simulink model "CMOS_Kernel_Memory_Sync"  (R2023b)
settings: Solver=VariableStepAuto  StartTime=0.0  StopTime=30000000  RelTol=1e-3
values from neighbouring files (symbols this model uses):
  AmountOfPixelsPerScanline = 400    [Kernel_Setup_Script.m]
  AmountOfRamBlocksScanlines = 5    [Kernel_Setup_Script.m]
  AmountOfRamBlocksScanlinesOffset = AmountOfRamBlocksScanlines - 1    (= 4)    [Kernel_Setup_Script.m]
  AmountOfScanlinePixels = 73700    [Kernel_Setup_Script.m]
  AmountOfScanlinePixelsOffset = AmountOfScanlinePixels - 1    (= 73699)    [Kernel_Setup_Script.m]
  AmountOfScanlines = 1100    [Kernel_Setup_Script.m]
  AmountOfScanlinesOffset = AmountOfScanlines - 1    (= 1099)    [Kernel_Setup_Script.m]
  AOPPK_Off = AmountOfPixelsPerScanline - 1    (= 399)    [Kernel_Setup_Script.m]
  AOPPS_Off = AmountOfPixelsPerScanline - 1    (= 399)    [Kernel_Setup_Script.m]
  FramePackOff_0 = FramePackOff_0 - ScanlineFifoCheck    [Kernel_Setup_Script.m]
  FramePackOff_1 = FramePackOff_1 - ScanlineFifoCheck    [Kernel_Setup_Script.m]
  FramePackOff_2 = FramePackOff_2 - ScanlineFifoCheck    [Kernel_Setup_Script.m]
  FramePackOff_3 = FramePackOff_3 - ScanlineFifoCheck    [Kernel_Setup_Script.m]
  FramePackOff_4 = FramePackOff_4 - ScanlineFifoCheck    [Kernel_Setup_Script.m]
  FramePackOff_5 = FramePackOff_5 - ScanlineFifoCheck    [Kernel_Setup_Script.m]
  KernelPackOff_0 = KernelPackOff_0 - KernelBitsPerRow    [Kernel_Setup_Script.m]
  KernelPackOff_1 = KernelPackOff_1 - KernelBitsPerRow    [Kernel_Setup_Script.m]
  KernelPackOff_2 = KernelPackOff_2 - KernelBitsPerRow    [Kernel_Setup_Script.m]
  KernelPackOff_3 = KernelPackOff_3 - KernelBitsPerRow    [Kernel_Setup_Script.m]
  Slice59DownTo48Top = (MsbOffset - (ScanlinePixelBitSizeController*1))    (= 59)    [Kernel_Setup_Script.m]
  Slice71DownTo60Top = (MsbOffset - (ScanlinePixelBitSizeController*0))    (= 71)    [Kernel_Setup_Script.m]
  TotalSectionsForFrames = AmountOfScanlines/AmountOfRamBlocksScanlines    (= 220)    [Kernel_Setup_Script.m]
  UltraRamRows = AmountOfPixelsPerScanline/ScanlineFifoCheck    [Kernel_Setup_Script.m]
  UltraRamRowsCeil = ceil(AmountOfPixelsPerScanline/ScanlineFifoCheck)    [Kernel_Setup_Script.m]
  UltraRamRowsKernel = AmountOfPixelsPerScanline/KernelBitsPerRow    (= 100)    [Kernel_Setup_Script.m]
  UltraRamRowsKernelCeil = ceil(AmountOfPixelsPerScanline/KernelBitsPerRow)    [Kernel_Setup_Script.m]
  UltraRamRowsMemorySectionOffset = UltraRamRowsCeil*AmountOfRamBlocksScanlines    [Kernel_Setup_Script.m]
  UltraRamRowsOffset = UltraRamRowsCeil - 1    [Kernel_Setup_Script.m]
undefined symbols (not defined in the file or in its folder): c, Down, sfvc784, Up, xck26
libraries: hdlBasic x4512, vmcUtilities x1
(part 3 of 39)

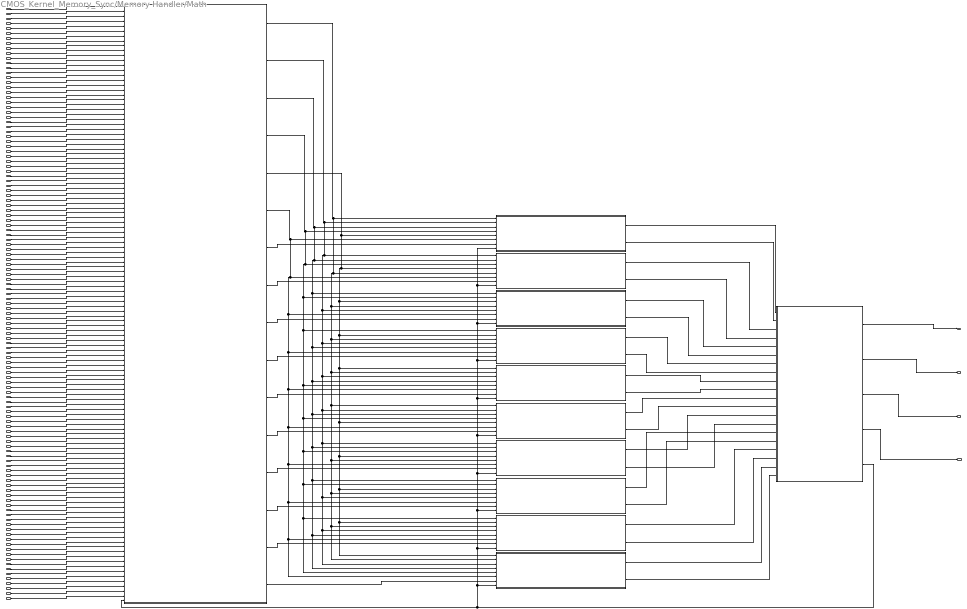
== system CMOS_Kernel_Memory_Sync/Memory Handler/Math ==
  In Pixel 0 at Offset 0 : Inport
  In Pixel 1 at Offset 0 : Inport  Port=2
  In Pixel 2 at Offset 0 : Inport  Port=3
  In Pixel 3 at Offset 0 : Inport  Port=4
  In Pixel 4 at Offset 0 : Inport  Port=5
  In Pixel 5 at Offset 0 : Inport  Port=6
  In Pixel 6 at Offset 0 : Inport  Port=7
  In Pixel 7 at Offset 0 : Inport  Port=8
  In Pixel 8 at Offset 0 : Inport  Port=9
  In Pixel 9 at Offset 0 : Inport  Port=10
  In Pixel 10 at Offset 0 : Inport  Port=11
  In Pixel 11 at Offset 0 : Inport  Port=12
  In Pixel 0 at Offset 1 : Inport  Port=13
  In Pixel 1 at Offset 1 : Inport  Port=14
  In Pixel 2 at Offset 1 : Inport  Port=15
  In Pixel 3 at Offset 1 : Inport  Port=16
  In Pixel 4 at Offset 1 : Inport  Port=17
  In Pixel 5 at Offset 1 : Inport  Port=18
  In Pixel 6 at Offset 1 : Inport  Port=19
  In Pixel 7 at Offset 1 : Inport  Port=20
  In Pixel 8 at Offset 1 : Inport  Port=21
  In Pixel 9 at Offset 1 : Inport  Port=22
  In Pixel 10 at Offset 1 : Inport  Port=23
  In Pixel 11 at Offset 1 : Inport  Port=24
  In Pixel 0 at Offset 2 : Inport  Port=25
  In Pixel 1 at Offset 2 : Inport  Port=26
  In Pixel 2 at Offset 2 : Inport  Port=27
  In Pixel 3 at Offset 2 : Inport  Port=28
  In Pixel 4 at Offset 2 : Inport  Port=29
  In Pixel 5 at Offset 2 : Inport  Port=30
  In Pixel 6 at Offset 2 : Inport  Port=31
  In Pixel 7 at Offset 2 : Inport  Port=32
  In Pixel 8 at Offset 2 : Inport  Port=33
  In Pixel 9 at Offset 2 : Inport  Port=34
  In Pixel 10 at Offset 2 : Inport  Port=35
  In Pixel 11 at Offset 2 : Inport  Port=36
  In Pixel 0 at Offset 3 : Inport  Port=37
  In Pixel 1 at Offset 3 : Inport  Port=38
  In Pixel 2 at Offset 3 : Inport  Port=39
  In Pixel 3 at Offset 3 : Inport  Port=40
  In Pixel 4 at Offset 3 : Inport  Port=41
  In Pixel 5 at Offset 3 : Inport  Port=42
  In Pixel 6 at Offset 3 : Inport  Port=43
  In Pixel 7 at Offset 3 : Inport  Port=44
  In Pixel 8 at Offset 3 : Inport  Port=45
  In Pixel 9 at Offset 3 : Inport  Port=46
  In Pixel 10 at Offset 3 : Inport  Port=47
  In Pixel 11 at Offset 3 : Inport  Port=48
  In Pixel 0 at Offset 4 : Inport  Port=49
  In Pixel 1 at Offset 4 : Inport  Port=50
  In Pixel 2 at Offset 4 : Inport  Port=51
  In Pixel 3 at Offset 4 : Inport  Port=52
  In Pixel 4 at Offset 4 : Inport  Port=53
  In Pixel 5 at Offset 4 : Inport  Port=54
  In Pixel 6 at Offset 4 : Inport  Port=55
  In Pixel 7 at Offset 4 : Inport  Port=56
  In Pixel 8 at Offset 4 : Inport  Port=57
  In Pixel 9 at Offset 4 : Inport  Port=58
  In Pixel 10 at Offset 4 : Inport  Port=59
  In Pixel 11 at Offset 4 : Inport  Port=60
  In Weight 0 at Offset 0 : Inport  Port=61
  In Weight 1 at Offset 0 : Inport  Port=62
  In Weight 2 at Offset 0 : Inport  Port=63
  In Weight 3 at Offset 0 : Inport  Port=64
  In Weight 4 at Offset 0 : Inport  Port=65
  In Weight 5 at Offset 0 : Inport  Port=66
  In Weight 6 at Offset 0 : Inport  Port=67
  In Weight 7 at Offset 0 : Inport  Port=68
  In Weight 8 at Offset 0 : Inport  Port=69
  In Weight 9 at Offset 0 : Inport  Port=70
  In Weight 10 at Offset 0 : Inport  Port=71
  In Weight 11 at Offset 0 : Inport  Port=72
  In Weight 0 at Offset 1 : Inport  Port=73
  In Weight 1 at Offset 1 : Inport  Port=74
  In Weight 2 at Offset 1 : Inport  Port=75
  In Weight 3 at Offset 1 : Inport  Port=76
  In Weight 4 at Offset 1 : Inport  Port=77
  In Weight 5 at Offset 1 : Inport  Port=78
  In Weight 6 at Offset 1 : Inport  Port=79
  In Weight 7 at Offset 1 : Inport  Port=80
  In Weight 8 at Offset 1 : Inport  Port=81
  In Weight 9 at Offset 1 : Inport  Port=82
  In Weight 10 at Offset 1 : Inport  Port=83
  In Weight 11 at Offset 1 : Inport  Port=84
  In Weight 0 at Offset 2 : Inport  Port=85
  In Weight 1 at Offset 2 : Inport  Port=86
  In Weight 2 at Offset 2 : Inport  Port=87
  In Weight 3 at Offset 2 : Inport  Port=88
  In Weight 4 at Offset 2 : Inport  Port=89
  In Weight 5 at Offset 2 : Inport  Port=90
  In Weight 6 at Offset 2 : Inport  Port=91
  In Weight 7 at Offset 2 : Inport  Port=92
  In Weight 8 at Offset 2 : Inport  Port=93
  In Weight 9 at Offset 2 : Inport  Port=94
  In Weight 10 at Offset 2 : Inport  Port=95
  In Weight 11 at Offset 2 : Inport  Port=96
  In Weight 0 at Offset 3 : Inport  Port=97
  In Weight 1 at Offset 3 : Inport  Port=98
  In Weight 2 at Offset 3 : Inport  Port=99
  In Weight 3 at Offset 3 : Inport  Port=100
  In Weight 4 at Offset 3 : Inport  Port=101
  In Weight 5 at Offset 3 : Inport  Port=102
  In Weight 6 at Offset 3 : Inport  Port=103
  In Weight 7 at Offset 3 : Inport  Port=104
  In Weight 8 at Offset 3 : Inport  Port=105
  In Weight 9 at Offset 3 : Inport  Port=106
  In Weight 10 at Offset 3 : Inport  Port=107
  In Weight 11 at Offset 3 : Inport  Port=108
  In Weight 0 at Offset 4 : Inport  Port=109
  In Weight 1 at Offset 4 : Inport  Port=110
  In Weight 2 at Offset 4 : Inport  Port=111
  In Weight 3 at Offset 4 : Inport  Port=112
  In Weight 4 at Offset 4 : Inport  Port=113
  In Weight 5 at Offset 4 : Inport  Port=114
  In Weight 6 at Offset 4 : Inport  Port=115
  In Weight 7 at Offset 4 : Inport  Port=116
  In Weight 8 at Offset 4 : Inport  Port=117
  In Weight 9 at Offset 4 : Inport  Port=118
  In Weight 10 at Offset 4 : Inport  Port=119
  In Weight 11 at Offset 4 : Inport  Port=120
  Valid Data In : Inport  Port=121
  Kernel Organizer : Subsystem
  Kernel Result 0 : Subsystem
  Kernel Result 1 : Subsystem
  Kernel Result 2 : Subsystem
  Kernel Result 3 : Subsystem
  Kernel Result 4 : Subsystem
  Kernel Result 5 : Subsystem
  Kernel Result 6 : Subsystem
  Kernel Result 7 : Subsystem
  Kernel Result 8 : Subsystem
  Kernel Result 9 : Subsystem
  Subsystem : Subsystem
  Kernel Output : Outport
  Valid Kernel Output : Outport  Port=2
  Kernel Result Array Position : Outport  Port=3
  Kernel Result Row Depth Position : Outport  Port=4
  wires:
  Kernel Organizer/1(Pixel Group Offset 0) -> Kernel Result 0/1(Pixel Bus Input Offset 0), Kernel Result 2/4(Pixel Bus Input Offset 3), Kernel Result 3/3(Pixel Bus Input Offset 2), Kernel Result 4/2(Pixel Bus Input Offset 1), Kernel Result 5/1(Pixel Bus Input Offset 0), Kernel Result 6/5(Pixel Bus Input Offset 4), Kernel Result 7/4(Pixel Bus Input Offset 3), Kernel Result 9/2(Pixel Bus Input Offset 1), Kernel Result 8/3(Pixel Bus Input Offset 2), Kernel Result 1/5(Pixel Bus Input Offset 4)
  Kernel Organizer/7(Kernel Result Valid Bus 0) -> Kernel Result 0/7(Valid Bus Input)
  Valid Data In/1 -> Kernel Organizer/121(Valid Data In)
  In Weight 11 at Offset 4/1 -> Kernel Organizer/120(In Weight 11 at Offset 4)
  In Weight 10 at Offset 4/1 -> Kernel Organizer/119(In Weight 10 at Offset 4)
  In Weight 9 at Offset 4/1 -> Kernel Organizer/118(In Weight 9 at Offset 4)
  In Weight 8 at Offset 4/1 -> Kernel Organizer/117(In Weight 8 at Offset 4)
  In Weight 7 at Offset 4/1 -> Kernel Organizer/116(In Weight 7 at Offset 4)
  In Weight 6 at Offset 4/1 -> Kernel Organizer/115(In Weight 6 at Offset 4)
  In Weight 5 at Offset 4/1 -> Kernel Organizer/114(In Weight 5 at Offset 4)
  In Weight 4 at Offset 4/1 -> Kernel Organizer/113(In Weight 4 at Offset 4)
  In Weight 3 at Offset 4/1 -> Kernel Organizer/112(In Weight 3 at Offset 4)
  In Weight 2 at Offset 4/1 -> Kernel Organizer/111(In Weight 2 at Offset 4)
  In Weight 1 at Offset 4/1 -> Kernel Organizer/110(In Weight 1 at Offset 4)
  In Weight 0 at Offset 4/1 -> Kernel Organizer/109(In Weight 0 at Offset 4)
  In Weight 11 at Offset 3/1 -> Kernel Organizer/108(In Weight 11 at Offset 3)
  In Weight 10 at Offset 3/1 -> Kernel Organizer/107(In Weight 10 at Offset 3)
  In Weight 9 at Offset 3/1 -> Kernel Organizer/106(In Weight 9 at Offset 3)
  In Weight 8 at Offset 3/1 -> Kernel Organizer/105(In Weight 8 at Offset 3)
  In Weight 7 at Offset 3/1 -> Kernel Organizer/104(In Weight 7 at Offset 3)
  In Weight 6 at Offset 3/1 -> Kernel Organizer/103(In Weight 6 at Offset 3)
  In Weight 5 at Offset 3/1 -> Kernel Organizer/102(In Weight 5 at Offset 3)
  In Weight 4 at Offset 3/1 -> Kernel Organizer/101(In Weight 4 at Offset 3)
  In Weight 3 at Offset 3/1 -> Kernel Organizer/100(In Weight 3 at Offset 3)
  In Weight 2 at Offset 3/1 -> Kernel Organizer/99(In Weight 2 at Offset 3)
  In Weight 1 at Offset 3/1 -> Kernel Organizer/98(In Weight 1 at Offset 3)
  In Weight 0 at Offset 3/1 -> Kernel Organizer/97(In Weight 0 at Offset 3)
  In Weight 6 at Offset 2/1 -> Kernel Organizer/91(In Weight 6 at Offset 2)
  In Weight 5 at Offset 1/1 -> Kernel Organizer/78(In Weight 5 at Offset 1)
  In Weight 6 at Offset 1/1 -> Kernel Organizer/79(In Weight 6 at Offset 1)
  In Weight 5 at Offset 2/1 -> Kernel Organizer/90(In Weight 5 at Offset 2)
  In Weight 7 at Offset 1/1 -> Kernel Organizer/80(In Weight 7 at Offset 1)
  In Weight 8 at Offset 2/1 -> Kernel Organizer/93(In Weight 8 at Offset 2)
  In Weight 1 at Offset 2/1 -> Kernel Organizer/86(In Weight 1 at Offset 2)
  In Weight 1 at Offset 1/1 -> Kernel Organizer/74(In Weight 1 at Offset 1)
  In Weight 11 at Offset 2/1 -> Kernel Organizer/96(In Weight 11 at Offset 2)
  In Weight 10 at Offset 2/1 -> Kernel Organizer/95(In Weight 10 at Offset 2)
  In Weight 2 at Offset 1/1 -> Kernel Organizer/75(In Weight 2 at Offset 1)
  In Weight 9 at Offset 2/1 -> Kernel Organizer/94(In Weight 9 at Offset 2)
  In Weight 3 at Offset 2/1 -> Kernel Organizer/88(In Weight 3 at Offset 2)
  In Weight 8 at Offset 1/1 -> Kernel Organizer/81(In Weight 8 at Offset 1)
  In Weight 4 at Offset 1/1 -> Kernel Organizer/77(In Weight 4 at Offset 1)
  In Weight 0 at Offset 2/1 -> Kernel Organizer/85(In Weight 0 at Offset 2)
  In Weight 3 at Offset 1/1 -> Kernel Organizer/76(In Weight 3 at Offset 1)
  In Weight 10 at Offset 1/1 -> Kernel Organizer/83(In Weight 10 at Offset 1)
  In Weight 4 at Offset 2/1 -> Kernel Organizer/89(In Weight 4 at Offset 2)
  In Weight 9 at Offset 1/1 -> Kernel Organizer/82(In Weight 9 at Offset 1)
  In Weight 7 at Offset 2/1 -> Kernel Organizer/92(In Weight 7 at Offset 2)
  In Weight 11 at Offset 1/1 -> Kernel Organizer/84(In Weight 11 at Offset 1)
  In Weight 2 at Offset 2/1 -> Kernel Organizer/87(In Weight 2 at Offset 2)
  In Weight 6 at Offset 0/1 -> Kernel Organizer/67(In Weight 6 at Offset 0)
  In Pixel 5 at Offset 4/1 -> Kernel Organizer/54(In Pixel 5 at Offset 4)
  In Pixel 6 at Offset 4/1 -> Kernel Organizer/55(In Pixel 6 at Offset 4)
  In Weight 5 at Offset 0/1 -> Kernel Organizer/66(In Weight 5 at Offset 0)
  In Pixel 7 at Offset 4/1 -> Kernel Organizer/56(In Pixel 7 at Offset 4)
  In Weight 8 at Offset 0/1 -> Kernel Organizer/69(In Weight 8 at Offset 0)
  In Weight 1 at Offset 0/1 -> Kernel Organizer/62(In Weight 1 at Offset 0)
  In Pixel 1 at Offset 4/1 -> Kernel Organizer/50(In Pixel 1 at Offset 4)
  In Weight 11 at Offset 0/1 -> Kernel Organizer/72(In Weight 11 at Offset 0)
  In Weight 10 at Offset 0/1 -> Kernel Organizer/71(In Weight 10 at Offset 0)
  In Pixel 2 at Offset 4/1 -> Kernel Organizer/51(In Pixel 2 at Offset 4)
  In Weight 9 at Offset 0/1 -> Kernel Organizer/70(In Weight 9 at Offset 0)
  In Weight 3 at Offset 0/1 -> Kernel Organizer/64(In Weight 3 at Offset 0)
  In Pixel 8 at Offset 4/1 -> Kernel Organizer/57(In Pixel 8 at Offset 4)
  In Pixel 4 at Offset 4/1 -> Kernel Organizer/53(In Pixel 4 at Offset 4)
  In Weight 0 at Offset 0/1 -> Kernel Organizer/61(In Weight 0 at Offset 0)
  In Weight 0 at Offset 1/1 -> Kernel Organizer/73(In Weight 0 at Offset 1)
  In Pixel 3 at Offset 4/1 -> Kernel Organizer/52(In Pixel 3 at Offset 4)
  In Pixel 10 at Offset 4/1 -> Kernel Organizer/59(In Pixel 10 at Offset 4)
  In Weight 4 at Offset 0/1 -> Kernel Organizer/65(In Weight 4 at Offset 0)
  In Pixel 9 at Offset 4/1 -> Kernel Organizer/58(In Pixel 9 at Offset 4)
  In Weight 7 at Offset 0/1 -> Kernel Organizer/68(In Weight 7 at Offset 0)
  In Pixel 11 at Offset 4/1 -> Kernel Organizer/60(In Pixel 11 at Offset 4)
  In Weight 2 at Offset 0/1 -> Kernel Organizer/63(In Weight 2 at Offset 0)
  In Pixel 6 at Offset 3/1 -> Kernel Organizer/43(In Pixel 6 at Offset 3)
  In Pixel 5 at Offset 2/1 -> Kernel Organizer/30(In Pixel 5 at Offset 2)
  In Pixel 1 at Offset 0/1 -> Kernel Organizer/2(In Pixel 1 at Offset 0)
  In Pixel 5 at Offset 3/1 -> Kernel Organizer/42(In Pixel 5 at Offset 3)
  In Pixel 7 at Offset 2/1 -> Kernel Organizer/32(In Pixel 7 at Offset 2)
  In Pixel 1 at Offset 3/1 -> Kernel Organizer/38(In Pixel 1 at Offset 3)
  In Pixel 1 at Offset 2/1 -> Kernel Organizer/26(In Pixel 1 at Offset 2)
  In Pixel 11 at Offset 3/1 -> Kernel Organizer/48(In Pixel 11 at Offset 3)
  In Pixel 10 at Offset 3/1 -> Kernel Organizer/47(In Pixel 10 at Offset 3)
  In Pixel 9 at Offset 3/1 -> Kernel Organizer/46(In Pixel 9 at Offset 3)
  In Pixel 0 at Offset 0/1 -> Kernel Organizer/1(In Pixel 0 at Offset 0)
  In Pixel 1 at Offset 1/1 -> Kernel Organizer/14(In Pixel 1 at Offset 1)
  In Pixel 4 at Offset 1/1 -> Kernel Organizer/17(In Pixel 4 at Offset 1)
  In Pixel 8 at Offset 1/1 -> Kernel Organizer/21(In Pixel 8 at Offset 1)
  In Pixel 3 at Offset 1/1 -> Kernel Organizer/16(In Pixel 3 at Offset 1)
  In Pixel 2 at Offset 1/1 -> Kernel Organizer/15(In Pixel 2 at Offset 1)
  In Pixel 8 at Offset 3/1 -> Kernel Organizer/45(In Pixel 8 at Offset 3)
  In Pixel 10 at Offset 1/1 -> Kernel Organizer/23(In Pixel 10 at Offset 1)
  In Pixel 9 at Offset 1/1 -> Kernel Organizer/22(In Pixel 9 at Offset 1)
  In Pixel 10 at Offset 0/1 -> Kernel Organizer/11(In Pixel 10 at Offset 0)
  In Pixel 3 at Offset 3/1 -> Kernel Organizer/40(In Pixel 3 at Offset 3)
  In Pixel 4 at Offset 2/1 -> Kernel Organizer/29(In Pixel 4 at Offset 2)
  In Pixel 7 at Offset 1/1 -> Kernel Organizer/20(In Pixel 7 at Offset 1)
  In Pixel 2 at Offset 2/1 -> Kernel Organizer/27(In Pixel 2 at Offset 2)
  In Pixel 11 at Offset 0/1 -> Kernel Organizer/12(In Pixel 11 at Offset 0)
  In Pixel 11 at Offset 1/1 -> Kernel Organizer/24(In Pixel 11 at Offset 1)
  In Pixel 8 at Offset 0/1 -> Kernel Organizer/9(In Pixel 8 at Offset 0)
  In Pixel 0 at Offset 1/1 -> Kernel Organizer/13(In Pixel 0 at Offset 1)
  In Pixel 8 at Offset 2/1 -> Kernel Organizer/33(In Pixel 8 at Offset 2)
  In Pixel 4 at Offset 0/1 -> Kernel Organizer/5(In Pixel 4 at Offset 0)
  In Pixel 5 at Offset 1/1 -> Kernel Organizer/18(In Pixel 5 at Offset 1)
  In Pixel 6 at Offset 2/1 -> Kernel Organizer/31(In Pixel 6 at Offset 2)
  In Pixel 5 at Offset 0/1 -> Kernel Organizer/6(In Pixel 5 at Offset 0)
  In Pixel 6 at Offset 0/1 -> Kernel Organizer/7(In Pixel 6 at Offset 0)
  In Pixel 3 at Offset 0/1 -> Kernel Organizer/4(In Pixel 3 at Offset 0)
  In Pixel 9 at Offset 0/1 -> Kernel Organizer/10(In Pixel 9 at Offset 0)
  In Pixel 7 at Offset 0/1 -> Kernel Organizer/8(In Pixel 7 at Offset 0)
  In Pixel 0 at Offset 2/1 -> Kernel Organizer/25(In Pixel 0 at Offset 2)
  In Pixel 2 at Offset 0/1 -> Kernel Organizer/3(In Pixel 2 at Offset 0)
  In Pixel 0 at Offset 3/1 -> Kernel Organizer/37(In Pixel 0 at Offset 3)
  In Pixel 0 at Offset 4/1 -> Kernel Organizer/49(In Pixel 0 at Offset 4)
  In Pixel 3 at Offset 2/1 -> Kernel Organizer/28(In Pixel 3 at Offset 2)
  In Pixel 10 at Offset 2/1 -> Kernel Organizer/35(In Pixel 10 at Offset 2)
  In Pixel 6 at Offset 1/1 -> Kernel Organizer/19(In Pixel 6 at Offset 1)
  In Pixel 4 at Offset 3/1 -> Kernel Organizer/41(In Pixel 4 at Offset 3)
  In Pixel 9 at Offset 2/1 -> Kernel Organizer/34(In Pixel 9 at Offset 2)
  In Pixel 7 at Offset 3/1 -> Kernel Organizer/44(In Pixel 7 at Offset 3)
  In Pixel 11 at Offset 2/1 -> Kernel Organizer/36(In Pixel 11 at Offset 2)
  In Pixel 2 at Offset 3/1 -> Kernel Organizer/39(In Pixel 2 at Offset 3)
  Kernel Organizer/2(Pixel Group Offset 1) -> Kernel Result 2/5(Pixel Bus Input Offset 4), Kernel Result 3/4(Pixel Bus Input Offset 3), Kernel Result 4/3(Pixel Bus Input Offset 2), Kernel Result 5/2(Pixel Bus Input Offset 1), Kernel Result 6/1(Pixel Bus Input Offset 0), Kernel Result 7/5(Pixel Bus Input Offset 4), Kernel Result 9/3(Pixel Bus Input Offset 2), Kernel Result 8/4(Pixel Bus Input Offset 3), Kernel Result 1/1(Pixel Bus Input Offset 0), Kernel Result 0/2(Pixel Bus Input Offset 1)
  Kernel Organizer/3(Pixel Group Offset 2) -> Kernel Result 2/1(Pixel Bus Input Offset 0), Kernel Result 3/5(Pixel Bus Input Offset 4), Kernel Result 4/4(Pixel Bus Input Offset 3), Kernel Result 5/3(Pixel Bus Input Offset 2), Kernel Result 6/2(Pixel Bus Input Offset 1), Kernel Result 7/1(Pixel Bus Input Offset 0), Kernel Result 9/4(Pixel Bus Input Offset 3), Kernel Result 8/5(Pixel Bus Input Offset 4), Kernel Result 1/2(Pixel Bus Input Offset 1), Kernel Result 0/3(Pixel Bus Input Offset 2)
  Kernel Organizer/4(Pixel Group Offset 3) -> Kernel Result 2/2(Pixel Bus Input Offset 1), Kernel Result 3/1(Pixel Bus Input Offset 0), Kernel Result 4/5(Pixel Bus Input Offset 4), Kernel Result 5/4(Pixel Bus Input Offset 3), Kernel Result 6/3(Pixel Bus Input Offset 2), Kernel Result 7/2(Pixel Bus Input Offset 1), Kernel Result 9/5(Pixel Bus Input Offset 4), Kernel Result 8/1(Pixel Bus Input Offset 0), Kernel Result 1/3(Pixel Bus Input Offset 2), Kernel Result 0/4(Pixel Bus Input Offset 3)
  Kernel Organizer/5(Pixel Group Offset 4) -> Kernel Result 2/3(Pixel Bus Input Offset 2), Kernel Result 3/2(Pixel Bus Input Offset 1), Kernel Result 4/1(Pixel Bus Input Offset 0), Kernel Result 5/5(Pixel Bus Input Offset 4), Kernel Result 6/4(Pixel Bus Input Offset 3), Kernel Result 7/3(Pixel Bus Input Offset 2), Kernel Result 9/1(Pixel Bus Input Offset 0), Kernel Result 8/2(Pixel Bus Input Offset 1), Kernel Result 1/4(Pixel Bus Input Offset 3), Kernel Result 0/5(Pixel Bus Input Offset 4)
  Kernel Organizer/6(Weights) -> Kernel Result 2/6(Weight Bus Input), Kernel Result 3/6(Weight Bus Input), Kernel Result 4/6(Weight Bus Input), Kernel Result 5/6(Weight Bus Input), Kernel Result 6/6(Weight Bus Input), Kernel Result 7/6(Weight Bus Input), Kernel Result 9/6(Weight Bus Input), Kernel Result 8/6(Weight Bus Input), Kernel Result 1/6(Weight Bus Input), Kernel Result 0/6(Weight Bus Input)
  Kernel Organizer/8(Kernel Result Valid Bus 1) -> Kernel Result 1/7(Valid Bus Input)
  Kernel Organizer/9(Kernel Result Valid Bus 2) -> Kernel Result 2/7(Valid Bus Input)
  Kernel Organizer/10(Kernel Result Valid Bus 3) -> Kernel Result 3/7(Valid Bus Input)
  Kernel Organizer/11(Kernel Result Valid Bus 4) -> Kernel Result 4/7(Valid Bus Input)
  Kernel Organizer/12(Kernel Result Valid Bus 5) -> Kernel Result 5/7(Valid Bus Input)
  Kernel Organizer/13(Kernel Result Valid Bus 6) -> Kernel Result 6/7(Valid Bus Input)
  Kernel Organizer/14(Kernel Result Valid Bus 7) -> Kernel Result 7/7(Valid Bus Input)
  Kernel Organizer/15(Kernel Result Valid Bus 8) -> Kernel Result 8/7(Valid Bus Input)
  Kernel Organizer/16(Kernel Result Valid Bus 9) -> Kernel Result 9/7(Valid Bus Input)
  Kernel Result 0/1(Kernel Output) -> Subsystem/1(Kernel Result 0)
  Kernel Result 0/2(Valid Kernel Output) -> Subsystem/2(Kernel Result Valid 0)
  Kernel Result 1/1(Kernel Output) -> Subsystem/3(Kernel Result 1)
  Kernel Result 1/2(Valid Kernel Output) -> Subsystem/4(Kernel Result Valid 1)
  Kernel Result 2/1(Kernel Output) -> Subsystem/5(Kernel Result 2)
  Kernel Result 2/2(Valid Kernel Output) -> Subsystem/6(Kernel Result Valid 2)
  Kernel Result 3/1(Kernel Output) -> Subsystem/7(Kernel Result 3)
  Kernel Result 3/2(Valid Kernel Output) -> Subsystem/8(Kernel Result Valid 3)
  Kernel Result 4/1(Kernel Output) -> Subsystem/9(Kernel Result 4)
  Kernel Result 4/2(Valid Kernel Output) -> Subsystem/10(Kernel Result Valid 4)
  Kernel Result 5/1(Kernel Output) -> Subsystem/11(Kernel Result 5)
  Kernel Result 5/2(Valid Kernel Output) -> Subsystem/12(Kernel Result Valid 5)
  Kernel Result 6/1(Kernel Output) -> Subsystem/13(Kernel Result 6)
  Kernel Result 6/2(Valid Kernel Output) -> Subsystem/14(Kernel Result Valid 6)
  Kernel Result 7/1(Kernel Output) -> Subsystem/15(Kernel Result 7)
  Kernel Result 7/2(Valid Kernel Output) -> Subsystem/16(Kernel Result Valid 7)
  Kernel Result 8/1(Kernel Output) -> Subsystem/17(Kernel Result 8)
  Kernel Result 8/2(Valid Kernel Output) -> Subsystem/18(Kernel Result Valid 8)
  Kernel Result 9/1(Kernel Output) -> Subsystem/19(Kernel Result 9)
  Kernel Result 9/2(Valid Kernel Output) -> Subsystem/20(Kernel Result Valid 9)
  Subsystem/1(Kernel Result Output) -> Kernel Output/1
  Subsystem/2(Kernel Result Output Valid) -> Valid Kernel Output/1
  Subsystem/4(Kernel Result Row Depth Position) -> Kernel Result Row Depth Position/1
  Subsystem/3(Kernel Result Array Position) -> Kernel Result Array Position/1
  Subsystem/5(Finished Cube) -> Kernel Result 9/8(Hard Reset), Kernel Result 8/8(Hard Reset), Kernel Result 7/8(Hard Reset), Kernel Result 6/8(Hard Reset), Kernel Result 5/8(Hard Reset), Kernel Result 4/8(Hard Reset), Kernel Result 3/8(Hard Reset), Kernel Result 2/8(Hard Reset), Kernel Result 1/8(Hard Reset), Kernel Result 0/8(Hard Reset), Kernel Organizer/122(Reset to Known State)

== system CMOS_Kernel_Memory_Sync/Memory Handler/Memory Manager ==
  12 Bit Spectrual Bin In : Inport
  Enable In Spectrual : Inport  Port=2
  18 Bit Kernel Data In : Inport  Port=3
  Enable In Kernel : Inport  Port=4
  Constant1 : hdlBasic/Constant  const=0  gui_display_data_type=Boolean  arith_type=Boolean  n_bits=1  bin_pt=0  preci_type=Single  exp_width=8  frac_width=24  explicit_period=off  period=1  XmcBlockStatus=1  maskContainerNames=tabcontainer1  block_type=constant  block_config=sysgen:Constant_config
  Frame Memory Controller : Subsystem
      settings: RTWMemSecFuncInitTerm=Inherit fRAM model  RTWMemSecFuncExecute=Inherit fRAM model  RTWMemSecDataConstants=Inherit fRAM model  RTWMemSecDataInternal=Inherit fRAM model  RTWMemSecDataParameters=Inherit fRAM model
  Kernel Memory Controller : Subsystem
      settings: RTWMemSecFuncInitTerm=Inherit fRAM model  RTWMemSecFuncExecute=Inherit fRAM model  RTWMemSecDataConstants=Inherit fRAM model  RTWMemSecDataInternal=Inherit fRAM model  RTWMemSecDataParameters=Inherit fRAM model
  Kernel Memory Subsystem : Subsystem
      settings: RTWMemSecFuncInitTerm=Inherit fRAM model  RTWMemSecFuncExecute=Inherit fRAM model  RTWMemSecDataConstants=Inherit fRAM model  RTWMemSecDataInternal=Inherit fRAM model  RTWMemSecDataParameters=Inherit fRAM model
  Memory Sync : Subsystem
      settings: RTWMemSecFuncInitTerm=Inherit fRAM model  RTWMemSecFuncExecute=Inherit fRAM model  RTWMemSecDataConstants=Inherit fRAM model  RTWMemSecDataInternal=Inherit fRAM model  RTWMemSecDataParameters=Inherit fRAM model
  Memory Sync Delay Frame Write : Subsystem
      settings: RTWMemSecFuncInitTerm=Inherit fRAM model  RTWMemSecFuncExecute=Inherit fRAM model  RTWMemSecDataConstants=Inherit fRAM model  RTWMemSecDataInternal=Inherit fRAM model  RTWMemSecDataParameters=Inherit fRAM model
  Memory Sync Delay Frame Write1 : Subsystem
      settings: RTWMemSecFuncInitTerm=Inherit fRAM model  RTWMemSecFuncExecute=Inherit fRAM model  RTWMemSecDataConstants=Inherit fRAM model  RTWMemSecDataInternal=Inherit fRAM model  RTWMemSecDataParameters=Inherit fRAM model
  Scanline Memory Subsystem : Subsystem
      settings: RTWMemSecFuncInitTerm=Inherit fRAM model  RTWMemSecFuncExecute=Inherit fRAM model  RTWMemSecDataConstants=Inherit fRAM model  RTWMemSecDataInternal=Inherit fRAM model  RTWMemSecDataParameters=Inherit fRAM model
  Spectrual RAM 0 Out : Outport
  Spectrual RAM 1 Out : Outport  Port=2
  Spectrual RAM 2 Out : Outport  Port=3
  Spectrual RAM 3 Out : Outport  Port=4
  Spectrual RAM 4 Out : Outport  Port=5
  Spectrual Valid : Outport  Port=6
  Kernel RAM 0 Out1 : Outport  Port=7
  Kernel RAM 1 Out1 : Outport  Port=8
  Kernel RAM 2 Out1 : Outport  Port=9
  Kernel RAM 3 Out1 : Outport  Port=10
  Kernel RAM 4 Out1 : Outport  Port=11
  " Kernel Valid" : Outport  Port=12
  wires:
  Scanline Memory Subsystem/1(RAM 0 Out) -> Spectrual RAM 0 Out/1
  Scanline Memory Subsystem/2(RAM 1 Out) -> Spectrual RAM 1 Out/1
  Enable In Kernel/1 -> Kernel Memory Controller/2(Enable In)
  12 Bit Spectrual Bin In/1 -> Frame Memory Controller/1(12 Bit Data In)
  Enable In Spectrual/1 -> Frame Memory Controller/2(Enable In)
  Scanline Memory Subsystem/4(RAM 3 Out) -> Spectrual RAM 3 Out/1
  Kernel Memory Subsystem/2(RAM 1 Out) -> Kernel RAM 1 Out1/1
  Scanline Memory Subsystem/6(Valid) -> Spectrual Valid/1
  Kernel Memory Subsystem/5(RAM 4 Out) -> Kernel RAM 4 Out1/1
  Kernel Memory Subsystem/4(RAM 3 Out) -> Kernel RAM 3 Out1/1
  Kernel Memory Subsystem/3(RAM 2 Out) -> Kernel RAM 2 Out1/1
  Kernel Memory Subsystem/6(Valid) -> " Kernel Valid"/1
  18 Bit Kernel Data In/1 -> Kernel Memory Controller/1(18 Bit Data In)
  Scanline Memory Subsystem/3(RAM 2 Out) -> Spectrual RAM 2 Out/1
  Scanline Memory Subsystem/5(RAM 4 Out) -> Spectrual RAM 4 Out/1
  Kernel Memory Subsystem/1(RAM 0 Out) -> Kernel RAM 0 Out1/1
  Frame Memory Controller/5(Memory Is Full) -> Memory Sync/1(Frame Memory Full)
  Frame Memory Controller/6(New Frame Finished) -> Memory Sync/3(New Frame)
  Constant1/1 -> Memory Sync/4(Reset)
  Kernel Memory Controller/5(Memory Is Full) -> Memory Sync/2(Kernel Memory Full)
  Memory Sync/1(Frame Memory Address) -> Scanline Memory Subsystem/1(Read Address)
  Memory Sync/2(Frame Read Enable) -> Scanline Memory Subsystem/2(Read Enable)
  Memory Sync/3(Kernel Memory Address) -> Kernel Memory Subsystem/1(Read Address)
  Memory Sync/4(Kernel Read Enable) -> Kernel Memory Subsystem/2(Read Enable)
  Frame Memory Controller/1(Data Out 72 Bits) -> Memory Sync Delay Frame Write/1(Data Out 72 Bits)
  Frame Memory Controller/2(Data Out Ready) -> Memory Sync Delay Frame Write/2(Data Out Ready)
  Frame Memory Controller/3(Data Address Out) -> Memory Sync Delay Frame Write/3(Data Address Out)
  Frame Memory Controller/4(Ram Bloack Sel Out) -> Memory Sync Delay Frame Write/4(Ram Bloack Sel Out)
  Memory Sync Delay Frame Write/1(Data To Write) -> Scanline Memory Subsystem/5(Data To Write)
  Memory Sync Delay Frame Write/2(Write Enable) -> Scanline Memory Subsystem/6(Write Enable)
  Memory Sync Delay Frame Write/3(Write Address) -> Scanline Memory Subsystem/3(Write Address)
  Memory Sync Delay Frame Write/4(Write Data to RAM Sel) -> Scanline Memory Subsystem/4(Write Data to RAM Sel)
  Kernel Memory Controller/1(Data Out 72 Bits) -> Memory Sync Delay Frame Write1/1(Data Out 72 Bits)
  Kernel Memory Controller/2(Data Out Ready) -> Memory Sync Delay Frame Write1/2(Data Out Ready)
  Kernel Memory Controller/3(Data Address Out) -> Memory Sync Delay Frame Write1/3(Data Address Out)
  Kernel Memory Controller/4(Ram Block Sel Out) -> Memory Sync Delay Frame Write1/4(Ram Bloack Sel Out)
  Memory Sync Delay Frame Write1/1(Data To Write) -> Kernel Memory Subsystem/5(Data To Write)
  Memory Sync Delay Frame Write1/2(Write Enable) -> Kernel Memory Subsystem/6(Write Enable)
  Memory Sync Delay Frame Write1/3(Write Address) -> Kernel Memory Subsystem/3(Write Address)
  Memory Sync Delay Frame Write1/4(Write Data to RAM Sel) -> Kernel Memory Subsystem/4(Write Data to RAM Sel)

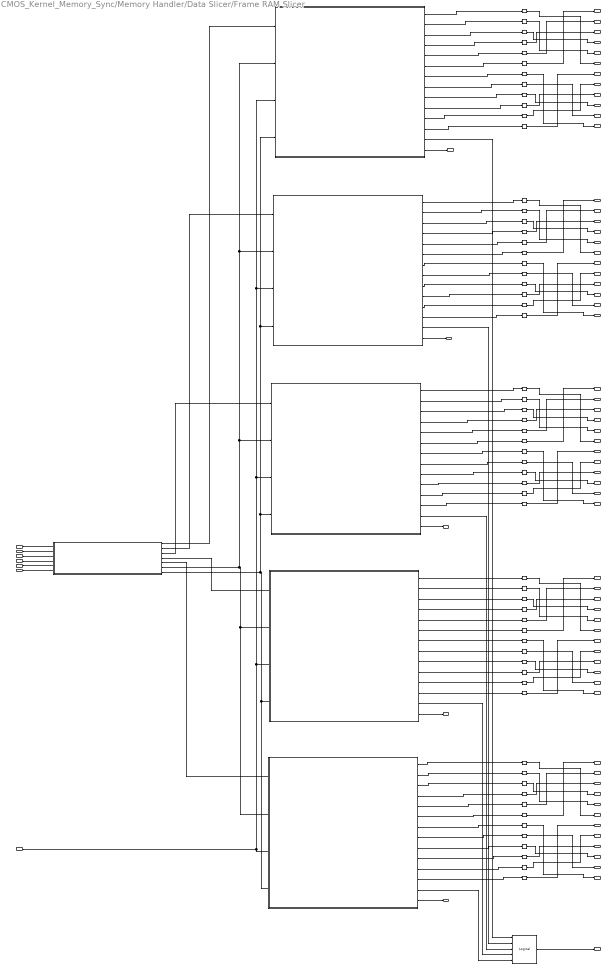
== system CMOS_Kernel_Memory_Sync/Memory Handler/Data Slicer/Frame RAM Slicer ==
  Data In RAM 0 : Inport
  Data In RAM 1 : Inport  Port=2
  Data In RAM 2 : Inport  Port=3
  Data In RAM 3 : Inport  Port=4
  Data In RAM 4 : Inport  Port=5
  Valid In : Inport  Port=6
  Read Enable : Inport  Port=7
  72 Bit Unpacker RAM 0 : Subsystem
      settings: RTWMemSecFuncInitTerm=Inherit fRAM model  RTWMemSecFuncExecute=Inherit fRAM model  RTWMemSecDataConstants=Inherit fRAM model  RTWMemSecDataInternal=Inherit fRAM model  RTWMemSecDataParameters=Inherit fRAM model
  72 Bit Unpacker RAM 1 : Subsystem
      settings: RTWMemSecFuncInitTerm=Inherit fRAM model  RTWMemSecFuncExecute=Inherit fRAM model  RTWMemSecDataConstants=Inherit fRAM model  RTWMemSecDataInternal=Inherit fRAM model  RTWMemSecDataParameters=Inherit fRAM model
  72 Bit Unpacker RAM 2 : Subsystem
      settings: RTWMemSecFuncInitTerm=Inherit fRAM model  RTWMemSecFuncExecute=Inherit fRAM model  RTWMemSecDataConstants=Inherit fRAM model  RTWMemSecDataInternal=Inherit fRAM model  RTWMemSecDataParameters=Inherit fRAM model
  72 Bit Unpacker RAM 3 : Subsystem
      settings: RTWMemSecFuncInitTerm=Inherit fRAM model  RTWMemSecFuncExecute=Inherit fRAM model  RTWMemSecDataConstants=Inherit fRAM model  RTWMemSecDataInternal=Inherit fRAM model  RTWMemSecDataParameters=Inherit fRAM model
  72 Bit Unpacker RAM 4 : Subsystem
      settings: RTWMemSecFuncInitTerm=Inherit fRAM model  RTWMemSecFuncExecute=Inherit fRAM model  RTWMemSecDataConstants=Inherit fRAM model  RTWMemSecDataInternal=Inherit fRAM model  RTWMemSecDataParameters=Inherit fRAM model
  Data Point Tracker : Subsystem
  Delay {0..51,60,65..71} (60 alike) : hdlBasic/Delay  rst=off  en=off  latency=1  reg_retiming=off  XmcBlockStatus=1  maskContainerNames=group1  block_type=delay  block_config=sysgen:Delay_config
  Valid Sync : hdlBasic/Logical  logical_function=AND  inputs=5  en=off  latency=1  precision=Full  arith_type=Unsigned  n_bits=16  bin_pt=0  align_bp=on  overflow=[]  quantization=[]  XmcBlockStatus=1  maskContainerNames=tabcontainer1  block_type=logical  block_config=sysgen:Logical_config
  Frame 12 Bit Bin Value 0 RAM 0 : Outport
  Frame 12 Bit Bin Value 1 RAM 0 : Outport  Port=2
  Frame 12 Bit Bin Value 2 RAM 0 : Outport  Port=3
  Frame 12 Bit Bin Value 3 RAM 0 : Outport  Port=4
  Frame 12 Bit Bin Value 4 RAM 0 : Outport  Port=5
  Frame 12 Bit Bin Value 5 RAM 0 : Outport  Port=6
  Frame 12 Bit Bin Value 6 RAM 0 : Outport  Port=7
  Frame 12 Bit Bin Value 7 RAM 0 : Outport  Port=8
  Frame 12 Bit Bin Value 8 RAM 0 : Outport  Port=9
  Frame 12 Bit Bin Value 9 RAM 0 : Outport  Port=10
  Frame 12 Bit Bin Value 10 RAM 0 : Outport  Port=11
  Frame 12 Bit Bin Value 11 RAM 0 : Outport  Port=12
  Frame 12 Bit Bin Value 0 RAM 1 : Outport  Port=13
  Frame 12 Bit Bin Value 1 RAM 1 : Outport  Port=14
  Frame 12 Bit Bin Value 2 RAM 1 : Outport  Port=15
  Frame 12 Bit Bin Value 3 RAM 1 : Outport  Port=16
  Frame 12 Bit Bin Value 4 RAM 1 : Outport  Port=17
  Frame 12 Bit Bin Value 5 RAM 1 : Outport  Port=18
  Frame 12 Bit Bin Value 6 RAM 1 : Outport  Port=19
  Frame 12 Bit Bin Value 7 RAM 1 : Outport  Port=20
  Frame 12 Bit Bin Value 8 RAM 1 : Outport  Port=21
  Frame 12 Bit Bin Value 9 RAM 1 : Outport  Port=22
  Frame 12 Bit Bin Value 10 RAM 1 : Outport  Port=23
  Frame 12 Bit Bin Value 11 RAM 1 : Outport  Port=24
  Frame 12 Bit Bin Value 0 RAM 2 : Outport  Port=25
  Frame 12 Bit Bin Value 1 RAM 2 : Outport  Port=26
  Frame 12 Bit Bin Value 2 RAM 2 : Outport  Port=27
  Frame 12 Bit Bin Value 3 RAM 2 : Outport  Port=28
  Frame 12 Bit Bin Value 4 RAM 2 : Outport  Port=29
  Frame 12 Bit Bin Value 5 RAM 2 : Outport  Port=30
  Frame 12 Bit Bin Value 6 RAM 2 : Outport  Port=31
  Frame 12 Bit Bin Value 7 RAM 2 : Outport  Port=32
  Frame 12 Bit Bin Value 8 RAM 2 : Outport  Port=33
  Frame 12 Bit Bin Value 9 RAM 2 : Outport  Port=34
  Frame 12 Bit Bin Value 10 RAM 2 : Outport  Port=35
  Frame 12 Bit Bin Value 11 RAM 2 : Outport  Port=36
  Frame 12 Bit Bin Value 0 RAM 3 : Outport  Port=37
  Frame 12 Bit Bin Value 1 RAM 3 : Outport  Port=38
  Frame 12 Bit Bin Value 2 RAM 3 : Outport  Port=39
  Frame 12 Bit Bin Value 3 RAM 3 : Outport  Port=40
  Frame 12 Bit Bin Value 4 RAM 3 : Outport  Port=41
  Frame 12 Bit Bin Value 5 RAM 3 : Outport  Port=42
  Frame 12 Bit Bin Value 6 RAM 3 : Outport  Port=43
  Frame 12 Bit Bin Value 7 RAM 3 : Outport  Port=44
  Frame 12 Bit Bin Value 8 RAM 3 : Outport  Port=45
  Frame 12 Bit Bin Value 9 RAM 3 : Outport  Port=46
  Frame 12 Bit Bin Value 10 RAM 3 : Outport  Port=47
  Frame 12 Bit Bin Value 11 RAM 3 : Outport  Port=48
  Frame 12 Bit Bin Value 0 RAM 4 : Outport  Port=49
  Frame 12 Bit Bin Value 1 RAM 4 : Outport  Port=50
  Frame 12 Bit Bin Value 2 RAM 4 : Outport  Port=51
  Frame 12 Bit Bin Value 3 RAM 4 : Outport  Port=52
  Frame 12 Bit Bin Value 4 RAM 4 : Outport  Port=53
  Frame 12 Bit Bin Value 5 RAM 4 : Outport  Port=54
  Frame 12 Bit Bin Value 6 RAM 4 : Outport  Port=55
  Frame 12 Bit Bin Value 7 RAM 4 : Outport  Port=56
  Frame 12 Bit Bin Value 8 RAM 4 : Outport  Port=57
  Frame 12 Bit Bin Value 9 RAM 4 : Outport  Port=58
  Frame 12 Bit Bin Value 10 RAM 4 : Outport  Port=59
  Frame 12 Bit Bin Value 11 RAM 4 : Outport  Port=60
  Valid Out : Outport  Port=61
  Wrote to Last FIFO RAM 0 : Outport  Port=62
  Wrote to Last FIFO RAM 1 : Outport  Port=63
  Wrote to Last FIFO RAM 2 : Outport  Port=64
  Wrote to Last FIFO RAM 3 : Outport  Port=65
  Wrote to Last FIFO RAM 4 : Outport  Port=66
  wires:
  72 Bit Unpacker RAM 0/6(11 Downto 0 FIFO 0) -> Delay 5/1
  72 Bit Unpacker RAM 0/5(23 Downto 12 FIFO 0) -> Delay 4/1
  72 Bit Unpacker RAM 0/4(35 Downto 24 FIFO 0) -> Delay 3/1
  72 Bit Unpacker RAM 0/3(47 Downto 36 FIFO 0) -> Delay 2/1
  72 Bit Unpacker RAM 0/2(59 Downto 48 FIFO 0) -> Delay 1/1
  72 Bit Unpacker RAM 0/1(71 Downto 60 FIFO 0) -> Delay 0/1
  72 Bit Unpacker RAM 0/12(11 Downto 0 FIFO 1) -> Delay 11/1
  72 Bit Unpacker RAM 0/11(23 Downto 12 FIFO 1) -> Delay 10/1
  72 Bit Unpacker RAM 0/10(35 Downto 24 FIFO 1) -> Delay 9/1
  72 Bit Unpacker RAM 0/9(47 Downto 36 FIFO 1) -> Delay 8/1
  72 Bit Unpacker RAM 0/8(59 Downto 48 FIFO 1) -> Delay 7/1
  72 Bit Unpacker RAM 0/7(71 Downto 60 FIFO 1) -> Delay 6/1
  Delay 0/1 -> Frame 12 Bit Bin Value 5 RAM 0/1
  Delay 1/1 -> Frame 12 Bit Bin Value 4 RAM 0/1
  Delay 2/1 -> Frame 12 Bit Bin Value 3 RAM 0/1
  Delay 3/1 -> Frame 12 Bit Bin Value 2 RAM 0/1
  Delay 4/1 -> Frame 12 Bit Bin Value 1 RAM 0/1
  Delay 5/1 -> Frame 12 Bit Bin Value 0 RAM 0/1
  Delay 6/1 -> Frame 12 Bit Bin Value 11 RAM 0/1
  Delay 7/1 -> Frame 12 Bit Bin Value 10 RAM 0/1
  Delay 8/1 -> Frame 12 Bit Bin Value 9 RAM 0/1
  Delay 9/1 -> Frame 12 Bit Bin Value 8 RAM 0/1
  Delay 10/1 -> Frame 12 Bit Bin Value 7 RAM 0/1
  Delay 11/1 -> Frame 12 Bit Bin Value 6 RAM 0/1
  72 Bit Unpacker RAM 1/7(71 Downto 60 FIFO 1) -> Delay 20/1
  72 Bit Unpacker RAM 1/10(35 Downto 24 FIFO 1) -> Delay 23/1
  72 Bit Unpacker RAM 1/8(59 Downto 48 FIFO 1) -> Delay 21/1
  72 Bit Unpacker RAM 1/4(35 Downto 24 FIFO 0) -> Delay 17/1
  72 Bit Unpacker RAM 1/12(11 Downto 0 FIFO 1) -> Delay 15/1
  Delay 12/1 -> Frame 12 Bit Bin Value 5 RAM 1/1
  72 Bit Unpacker RAM 1/1(71 Downto 60 FIFO 0) -> Delay 12/1
  72 Bit Unpacker RAM 1/6(11 Downto 0 FIFO 0) -> Delay 19/1
  72 Bit Unpacker RAM 1/11(23 Downto 12 FIFO 1) -> Delay 14/1
  72 Bit Unpacker RAM 1/2(59 Downto 48 FIFO 0) -> Delay 13/1
  Delay 22/1 -> Frame 12 Bit Bin Value 9 RAM 1/1
  Delay 14/1 -> Frame 12 Bit Bin Value 7 RAM 1/1
  Delay 13/1 -> Frame 12 Bit Bin Value 4 RAM 1/1
  72 Bit Unpacker RAM 1/5(23 Downto 12 FIFO 0) -> Delay 18/1
  Delay 18/1 -> Frame 12 Bit Bin Value 1 RAM 1/1
  Delay 20/1 -> Frame 12 Bit Bin Value 11 RAM 1/1
  72 Bit Unpacker RAM 1/3(47 Downto 36 FIFO 0) -> Delay 16/1
  Delay 17/1 -> Frame 12 Bit Bin Value 2 RAM 1/1
  Delay 23/1 -> Frame 12 Bit Bin Value 8 RAM 1/1
  Delay 15/1 -> Frame 12 Bit Bin Value 6 RAM 1/1
  Delay 19/1 -> Frame 12 Bit Bin Value 0 RAM 1/1
  Delay 21/1 -> Frame 12 Bit Bin Value 10 RAM 1/1
  Delay 16/1 -> Frame 12 Bit Bin Value 3 RAM 1/1
  72 Bit Unpacker RAM 1/9(47 Downto 36 FIFO 1) -> Delay 22/1
  72 Bit Unpacker RAM 2/7(71 Downto 60 FIFO 1) -> Delay 44/1
  72 Bit Unpacker RAM 2/8(59 Downto 48 FIFO 1) -> Delay 45/1
  72 Bit Unpacker RAM 2/4(35 Downto 24 FIFO 0) -> Delay 41/1
  72 Bit Unpacker RAM 2/12(11 Downto 0 FIFO 1) -> Delay 27/1
  Delay 24/1 -> Frame 12 Bit Bin Value 5 RAM 2/1
  72 Bit Unpacker RAM 2/1(71 Downto 60 FIFO 0) -> Delay 24/1
  72 Bit Unpacker RAM 2/2(59 Downto 48 FIFO 0) -> Delay 25/1
  Delay 46/1 -> Frame 12 Bit Bin Value 9 RAM 2/1
  Delay 26/1 -> Frame 12 Bit Bin Value 7 RAM 2/1
  Delay 25/1 -> Frame 12 Bit Bin Value 4 RAM 2/1
  72 Bit Unpacker RAM 3/9(47 Downto 36 FIFO 1) -> Delay 39/1
  72 Bit Unpacker RAM 2/6(11 Downto 0 FIFO 0) -> Delay 43/1
  72 Bit Unpacker RAM 2/11(23 Downto 12 FIFO 1) -> Delay 26/1
  Delay 34/1 -> Frame 12 Bit Bin Value 1 RAM 3/1
  72 Bit Unpacker RAM 3/3(47 Downto 36 FIFO 0) -> Delay 32/1
  Delay 29/1 -> Frame 12 Bit Bin Value 4 RAM 3/1
  Delay 37/1 -> Frame 12 Bit Bin Value 11 RAM 3/1
  Delay 38/1 -> Frame 12 Bit Bin Value 10 RAM 3/1
  Delay 31/1 -> Frame 12 Bit Bin Value 6 RAM 3/1
  Delay 35/1 -> Frame 12 Bit Bin Value 0 RAM 3/1
  Delay 33/1 -> Frame 12 Bit Bin Value 2 RAM 3/1
  Delay 39/1 -> Frame 12 Bit Bin Value 9 RAM 3/1
  Delay 30/1 -> Frame 12 Bit Bin Value 7 RAM 3/1
  72 Bit Unpacker RAM 3/12(11 Downto 0 FIFO 1) -> Delay 31/1
  Delay 32/1 -> Frame 12 Bit Bin Value 3 RAM 3/1
  72 Bit Unpacker RAM 3/4(35 Downto 24 FIFO 0) -> Delay 33/1
  72 Bit Unpacker RAM 3/1(71 Downto 60 FIFO 0) -> Delay 28/1
  72 Bit Unpacker RAM 2/10(35 Downto 24 FIFO 1) -> Delay 47/1
  72 Bit Unpacker RAM 3/8(59 Downto 48 FIFO 1) -> Delay 38/1
  72 Bit Unpacker RAM 3/2(59 Downto 48 FIFO 0) -> Delay 29/1
  72 Bit Unpacker RAM 3/10(35 Downto 24 FIFO 1) -> Delay 40/1
  Delay 28/1 -> Frame 12 Bit Bin Value 5 RAM 3/1
  72 Bit Unpacker RAM 3/6(11 Downto 0 FIFO 0) -> Delay 35/1
  72 Bit Unpacker RAM 2/5(23 Downto 12 FIFO 0) -> Delay 42/1
  Delay 42/1 -> Frame 12 Bit Bin Value 1 RAM 2/1
  Delay 44/1 -> Frame 12 Bit Bin Value 11 RAM 2/1
  72 Bit Unpacker RAM 2/3(47 Downto 36 FIFO 0) -> Delay 36/1
  Delay 41/1 -> Frame 12 Bit Bin Value 2 RAM 2/1
  Delay 40/1 -> Frame 12 Bit Bin Value 8 RAM 3/1
  Delay 47/1 -> Frame 12 Bit Bin Value 8 RAM 2/1
  72 Bit Unpacker RAM 3/7(71 Downto 60 FIFO 1) -> Delay 37/1
  72 Bit Unpacker RAM 3/5(23 Downto 12 FIFO 0) -> Delay 34/1
  Delay 27/1 -> Frame 12 Bit Bin Value 6 RAM 2/1
  Delay 43/1 -> Frame 12 Bit Bin Value 0 RAM 2/1
  Delay 45/1 -> Frame 12 Bit Bin Value 10 RAM 2/1
  Delay 36/1 -> Frame 12 Bit Bin Value 3 RAM 2/1
  72 Bit Unpacker RAM 3/11(23 Downto 12 FIFO 1) -> Delay 30/1
  72 Bit Unpacker RAM 2/9(47 Downto 36 FIFO 1) -> Delay 46/1
  72 Bit Unpacker RAM 4/7(71 Downto 60 FIFO 1) -> Delay 68/1
  72 Bit Unpacker RAM 4/8(59 Downto 48 FIFO 1) -> Delay 69/1
  72 Bit Unpacker RAM 4/4(35 Downto 24 FIFO 0) -> Delay 65/1
  72 Bit Unpacker RAM 4/12(11 Downto 0 FIFO 1) -> Delay 51/1
  Delay 48/1 -> Frame 12 Bit Bin Value 5 RAM 4/1
  72 Bit Unpacker RAM 4/1(71 Downto 60 FIFO 0) -> Delay 48/1
  72 Bit Unpacker RAM 4/2(59 Downto 48 FIFO 0) -> Delay 49/1
  Delay 70/1 -> Frame 12 Bit Bin Value 9 RAM 4/1
  Delay 50/1 -> Frame 12 Bit Bin Value 7 RAM 4/1
  Delay 49/1 -> Frame 12 Bit Bin Value 4 RAM 4/1
  72 Bit Unpacker RAM 4/6(11 Downto 0 FIFO 0) -> Delay 67/1
  72 Bit Unpacker RAM 4/11(23 Downto 12 FIFO 1) -> Delay 50/1
  72 Bit Unpacker RAM 4/10(35 Downto 24 FIFO 1) -> Delay 71/1
  72 Bit Unpacker RAM 4/5(23 Downto 12 FIFO 0) -> Delay 66/1
  Delay 66/1 -> Frame 12 Bit Bin Value 1 RAM 4/1
  Delay 68/1 -> Frame 12 Bit Bin Value 11 RAM 4/1
  72 Bit Unpacker RAM 4/3(47 Downto 36 FIFO 0) -> Delay 60/1
  Delay 65/1 -> Frame 12 Bit Bin Value 2 RAM 4/1
  Delay 71/1 -> Frame 12 Bit Bin Value 8 RAM 4/1
  Delay 51/1 -> Frame 12 Bit Bin Value 6 RAM 4/1
  Delay 67/1 -> Frame 12 Bit Bin Value 0 RAM 4/1
  Delay 69/1 -> Frame 12 Bit Bin Value 10 RAM 4/1
  Delay 60/1 -> Frame 12 Bit Bin Value 3 RAM 4/1
  72 Bit Unpacker RAM 4/9(47 Downto 36 FIFO 1) -> Delay 70/1
  Valid Sync/1 -> Valid Out/1
  72 Bit Unpacker RAM 0/13(Valid Out) -> Valid Sync/1
  72 Bit Unpacker RAM 1/13(Valid Out) -> Valid Sync/2
  72 Bit Unpacker RAM 2/13(Valid Out) -> Valid Sync/3
  72 Bit Unpacker RAM 3/13(Valid Out) -> Valid Sync/4
  72 Bit Unpacker RAM 4/13(Valid Out) -> Valid Sync/5
  Read Enable/1 -> 72 Bit Unpacker RAM 4/3(Read Enable), 72 Bit Unpacker RAM 3/3(Read Enable), 72 Bit Unpacker RAM 2/3(Read Enable), 72 Bit Unpacker RAM 1/3(Read Enable), 72 Bit Unpacker RAM 0/3(Read Enable)
  Data Point Tracker/6(Valid Enable Out) -> 72 Bit Unpacker RAM 4/2(Enable), 72 Bit Unpacker RAM 3/2(Enable), 72 Bit Unpacker RAM 2/2(Enable), 72 Bit Unpacker RAM 1/2(Enable), 72 Bit Unpacker RAM 0/2(Enable)
  Data In RAM 0/1 -> Data Point Tracker/1(Data In RAM 0)
  Data In RAM 1/1 -> Data Point Tracker/2(Data In RAM 1)
  Data In RAM 2/1 -> Data Point Tracker/3(Data In RAM 2)
  Data In RAM 3/1 -> Data Point Tracker/4(Data In RAM 3)
  Data In RAM 4/1 -> Data Point Tracker/5(Data In RAM 4)
  Valid In/1 -> Data Point Tracker/6(Valid Enable In)
  Data Point Tracker/1(Data Out RAM 0) -> 72 Bit Unpacker RAM 0/1(Data In)
  Data Point Tracker/2(Data Out RAM 1) -> 72 Bit Unpacker RAM 1/1(Data In)
  Data Point Tracker/3(Data Out RAM 2) -> 72 Bit Unpacker RAM 2/1(Data In)
  Data Point Tracker/4(Data Out RAM 3) -> 72 Bit Unpacker RAM 3/1(Data In)
  Data Point Tracker/5(Data Out RAM 4) -> 72 Bit Unpacker RAM 4/1(Data In)
  Data Point Tracker/7(Last Value Out) -> 72 Bit Unpacker RAM 2/4(Last Point), 72 Bit Unpacker RAM 1/4(Last Point), 72 Bit Unpacker RAM 0/4(Last Point), 72 Bit Unpacker RAM 4/4(Last Point), 72 Bit Unpacker RAM 3/4(Last Point)
  72 Bit Unpacker RAM 0/14(Wrote To a FIFO) -> Wrote to Last FIFO RAM 0/1
  72 Bit Unpacker RAM 1/14(Wrote To a FIFO) -> Wrote to Last FIFO RAM 1/1
  72 Bit Unpacker RAM 2/14(Wrote To a FIFO) -> Wrote to Last FIFO RAM 2/1
  72 Bit Unpacker RAM 3/14(Wrote To a FIFO) -> Wrote to Last FIFO RAM 3/1
  72 Bit Unpacker RAM 4/14(Wrote To a FIFO) -> Wrote to Last FIFO RAM 4/1
